simulink model "Trot"  (R2025b)
settings: Solver=VariableStepAuto  StartTime=0.0  StopTime=60  RelTol=0.01  AbsTol=0.01  EnableMultiTasking=on
undefined symbols (not defined in the file): a, b, c, X, Y, Z
libraries: sm_lib x58, nesl_utility x37, hdlsllib x12
(part 3 of 4)

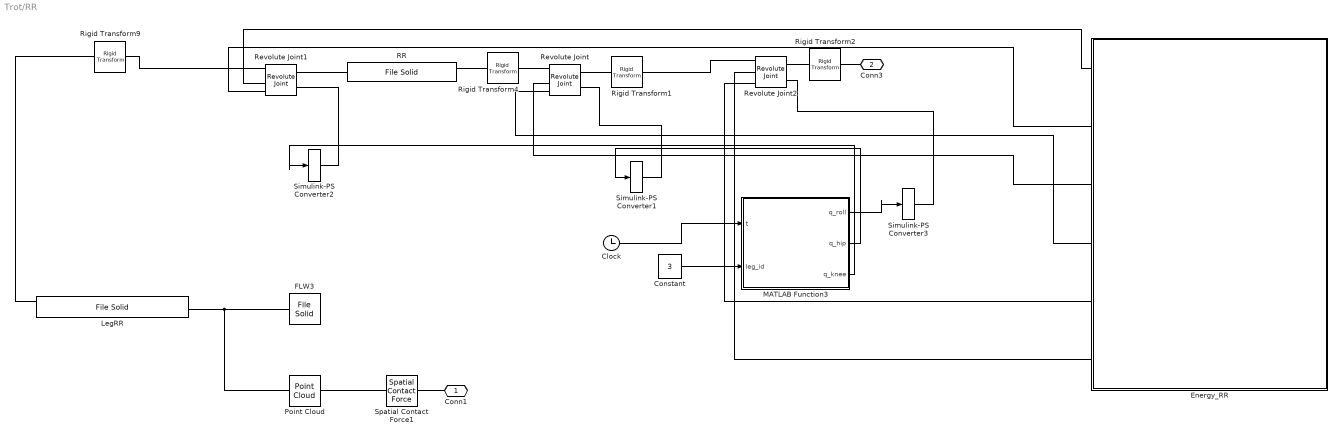
== system Trot/RR ==
  Clock : Clock
  Constant : Constant  Value=3
  Energy_RR : Subsystem
  FLW3 : sm_lib/Body Elements/File Solid  ExtGeomFileName=Cheng Shin C-166-1.stp  UnitType=FromFile  ExtGeomFileUnits=m  StepReaderType=HEX  ExportConvexHullGeometry=on  InertiaType=CalculateFromGeometry  BasedOnType=Density  Density=400  DensityUnits=kg/m^3  Mass=1  MassUnits=kg  CenterOfMass=[0 0 0]  CenterOfMassUnits=m  MomentsOfInertia=[1 1 1]  MomentsOfInertiaUnits=kg*m^2  ProductsOfInertia=[0 0 0]  ProductsOfInertiaUnits=kg*m^2  GraphicType=FromGeometry  MarkerShape=Sphere  MarkerSize=10  GraphicVisPropType=AdvancedVisualProperties  GraphicDiffuseColor=[0.1 0.1 0.1]  GraphicOpacity=1  GraphicSpecularColor=[0.2 0.2 0.2 1.0]  GraphicAmbientColor=[0.05 0.05 0.05 1.0]  GraphicEmissiveColor=[0.0 0.0 0.0 1.0]  GraphicShininess=10  DoExposeReferenceFrame=off  SerializedFrames=<Frames><Frame><Id>Frame1</Id><Value><Name>F1</Name><Origin><Source>CenterOfMassFrame</Source><FeatureName>toroidal surface 99</FeatureName></Origin><PrimaryAxis><DefinedDirection>+Z</DefinedDirection><Source>ReferenceFrame</Source><SourceDirection>+Z</SourceDirection><FeatureName></FeatureName></PrimaryAxis><SecondaryAxis><DefinedDirection>+X</DefinedDirection><Source>ReferenceFrame</Source><SourceDirection>+X</SourceDirection><FeatureName></FeatureName></SecondaryAxis></Value></Frame></Frames>
  LegRR : sm_lib/Body Elements/File Solid  ExtGeomFileName=leg.STEP  UnitType=FromFile  ExtGeomFileUnits=m  StepReaderType=HEX  ExportConvexHullGeometry=on  InertiaType=CalculateFromGeometry  BasedOnType=Density  Density=800  DensityUnits=kg/m^3  Mass=1  MassUnits=kg  CenterOfMass=[0 0 0]  CenterOfMassUnits=m  MomentsOfInertia=[1 1 1]  MomentsOfInertiaUnits=kg*m^2  ProductsOfInertia=[0 0 0]  ProductsOfInertiaUnits=kg*m^2  GraphicType=FromGeometry  MarkerShape=Sphere  MarkerSize=10  GraphicVisPropType=AdvancedVisualProperties  GraphicDiffuseColor=[0 0 0]  GraphicOpacity=1  GraphicSpecularColor=[0.9 0.9 0.9 1.0]  GraphicAmbientColor=[0.1 0.1 0.1 1.0]  GraphicEmissiveColor=[0.0 0.0 0.0 1.0]  GraphicShininess=100  DoExposeReferenceFrame=off  SerializedFrames=|
      | <Frames>
      | 
      |   <Frame>
      |     <Id>Frame1</Id>
      |     <Value>
      |       <Name>L-K link</Name>
      |       <Origin>
      |         <Source>GeometricFeature</Source>
      |         <FeatureName>cylindrical surface 6</FeatureName>
      |       </Origin>
      |       <PrimaryAxis>
      |         <DefinedDirection>+Z</DefinedDirection>
      |         <Source>ReferenceFrame</Source>
      |         <SourceDirection>+Z</SourceDirection>
      |         <FeatureName></FeatureName>
      |       </PrimaryAxis>
      |       <SecondaryAxis>
      |         <DefinedDirection>+X</DefinedDirection>
      |         <Source>ReferenceFrame</Source>
      |         <SourceDirection>-X</SourceDirection>
      |         <FeatureName></FeatureName>
      |       </SecondaryAxis>
      |     </Value>
      |   </Frame>
      | 
      |   <Frame>
      |     <Id>Frame2</Id>
      |     <Value>
      |       <Name>L-W link</Name>
      |       <Origin>
      |         <Source>GeometricFeature</Source>
      |         <FeatureName>cylindrical surface 4</FeatureName>
      |       </Origin>
      |       <PrimaryAxis>
      |         <DefinedDirection>+Z</DefinedDirection>
      |         <Source>ReferenceFrame</Source>
      |         <SourceDirection>+Z</SourceDirection>
      |         <FeatureName></FeatureName>
      |       </PrimaryAxis>
      |       <SecondaryAxis>
      |         <DefinedDirection>+X</DefinedDirection>
      |         <Source>ReferenceFrame</Source>
      |         <SourceDirection>-X</SourceDirection>
      |         <FeatureName></FeatureName>
      |       </SecondaryAxis>
      |     </Value>
      |   </Frame>
      | 
      | </Frames>
  MATLAB Function3 : MATLAB Function  TreatAsAtomicUnit=on
  Point Cloud : sm_lib/Curves and Surfaces/Point Cloud  CoordinatesMatrix=wheel_pts  CoordinatesMatrixUnits=m  GraphicType=MarkerCloud  GraphicSphereRadius=1e-2  GraphicSphereRadiusUnits=m  GraphicVisPropType=SimpleVisualProperties  GraphicDiffuseColor=[0.5 0.5 0.5]  GraphicOpacity=1  GraphicSpecularColor=[0.5 0.5 0.5 1.0]  GraphicAmbientColor=[0.15 0.15 0.15 1.0]  GraphicEmissiveColor=[0.0 0.0 0.0 1.0]  GraphicShininess=75
  RR : sm_lib/Body Elements/File Solid  ExtGeomFileName=haut patte D.STEP  UnitType=FromFile  ExtGeomFileUnits=m  StepReaderType=HEX  ExportConvexHullGeometry=on  InertiaType=CalculateFromGeometry  BasedOnType=Density  Density=800  DensityUnits=kg/m^3  Mass=1  MassUnits=kg  CenterOfMass=[0 0 0]  CenterOfMassUnits=m  MomentsOfInertia=[1 1 1]  MomentsOfInertiaUnits=kg*m^2  ProductsOfInertia=[0 0 0]  ProductsOfInertiaUnits=kg*m^2  GraphicType=FromGeometry  MarkerShape=Sphere  MarkerSize=10  GraphicVisPropType=AdvancedVisualProperties  GraphicDiffuseColor=[0.9 0.9 0.9]  GraphicOpacity=1  GraphicSpecularColor=[0.9 0.9 0.9 1.0]  GraphicAmbientColor=[0.1 0.1 0.1 1.0]  GraphicEmissiveColor=[0.0 0.0 0.0 1.0]  GraphicShininess=100  DoExposeReferenceFrame=off  SerializedFrames=<Frames><Frame><Id>Frame1</Id><Value><Name>H-L link</Name><Origin><Source>GeometricFeature</Source><FeatureName>spherical surface 2</FeatureName></Origin><PrimaryAxis><DefinedDirection>+Z</DefinedDirection><Source>ReferenceFrame</Source><SourceDirection>+Z</SourceDirection><FeatureName></FeatureName></PrimaryAxis><SecondaryAxis><DefinedDirection>+X</DefinedDirection><Source>ReferenceFrame</Source><SourceDirection>-Y</SourceDirection><FeatureName></FeatureName></SecondaryAxis></Value></Frame><Frame><Id>Frame2</Id><Value><Name>L-K link</Name><Origin><Source>GeometricFeature</Source><FeatureName>cylindrical surface 2</FeatureName></Origin><PrimaryAxis><DefinedDirection>+Z</DefinedDirection><Source>ReferenceFrame</Source><SourceDirection>+Z</SourceDirection><FeatureName></FeatureName></PrimaryAxis><SecondaryAxis><DefinedDirection>+X</DefinedDirection><Source>ReferenceFrame</Source><SourceDirection>-Y</SourceDirection><FeatureName></FeatureName></SecondaryAxis></Value></Frame></Frames>
  Revolute Joint : sm_lib/Joints/Revolute Joint  JointMode=Normal  CompositeWrenchDir=FollowerOnBase  CompositeWrenchFrame=BaseFrame  SenseConstraintForce=off  SenseConstraintTorque=off  SenseTotalForce=off  SenseTotalTorque=off  PositionTargetSpecify=off  PositionTargetPriority=High  PositionTargetValue=0  PositionTargetValueUnits=deg  VelocityTargetSpecify=off  VelocityTargetPriority=High  VelocityTargetValue=0  VelocityTargetValueUnits=deg/s  EquilibriumPosition=0  EquilibriumPositionUnits=deg  SpringStiffness=0  SpringStiffnessUnits=N*m/deg  DampingCoefficient=0  DampingCoefficientUnits=N*m/(deg/s)  LowerLimitSpecify=off  LowerLimitBound=-90  LowerLimitBoundUnits=deg  LowerLimitStiffness=1e4  LowerLimitStiffnessUnits=N*m/deg  LowerLimitDamping=10  LowerLimitDampingUnits=N*m/(deg/s)  LowerLimitTransitionRegionWidth=0.1  LowerLimitTransitionRegionWidthUnits=deg  UpperLimitSpecify=off  UpperLimitBound=90  UpperLimitBoundUnits=deg  UpperLimitStiffness=1e4  UpperLimitStiffnessUnits=N*m/deg  UpperLimitDamping=10  UpperLimitDampingUnits=N*m/(deg/s)  UpperLimitTransitionRegionWidth=0.1  UpperLimitTransitionRegionWidthUnits=deg  TorqueActuationMode=ComputedTorque  MotionActuationMode=InputMotion  SensePosition=on  SenseVelocity=on  SenseAcceleration=off  SenseTorqueForce=on  SenseLowerLimitTorqueForce=off  SenseUpperLimitTorqueForce=off
  Revolute Joint1 : sm_lib/Joints/Revolute Joint  JointMode=Normal  CompositeWrenchDir=FollowerOnBase  CompositeWrenchFrame=BaseFrame  SenseConstraintForce=off  SenseConstraintTorque=off  SenseTotalForce=off  SenseTotalTorque=off  PositionTargetSpecify=off  PositionTargetPriority=High  PositionTargetValue=0  PositionTargetValueUnits=deg  VelocityTargetSpecify=off  VelocityTargetPriority=High  VelocityTargetValue=0  VelocityTargetValueUnits=deg/s  EquilibriumPosition=0  EquilibriumPositionUnits=deg  SpringStiffness=0  SpringStiffnessUnits=N*m/deg  DampingCoefficient=0  DampingCoefficientUnits=N*m/(deg/s)  LowerLimitSpecify=off  LowerLimitBound=-90  LowerLimitBoundUnits=deg  LowerLimitStiffness=1e4  LowerLimitStiffnessUnits=N*m/deg  LowerLimitDamping=10  LowerLimitDampingUnits=N*m/(deg/s)  LowerLimitTransitionRegionWidth=0.1  LowerLimitTransitionRegionWidthUnits=deg  UpperLimitSpecify=off  UpperLimitBound=90  UpperLimitBoundUnits=deg  UpperLimitStiffness=1e4  UpperLimitStiffnessUnits=N*m/deg  UpperLimitDamping=10  UpperLimitDampingUnits=N*m/(deg/s)  UpperLimitTransitionRegionWidth=0.1  UpperLimitTransitionRegionWidthUnits=deg  TorqueActuationMode=ComputedTorque  MotionActuationMode=InputMotion  SensePosition=on  SenseVelocity=on  SenseAcceleration=off  SenseTorqueForce=on  SenseLowerLimitTorqueForce=off  SenseUpperLimitTorqueForce=off
  Revolute Joint2 : sm_lib/Joints/Revolute Joint  JointMode=Normal  CompositeWrenchDir=FollowerOnBase  CompositeWrenchFrame=BaseFrame  SenseConstraintForce=off  SenseConstraintTorque=off  SenseTotalForce=off  SenseTotalTorque=off  PositionTargetSpecify=off  PositionTargetPriority=High  PositionTargetValue=0  PositionTargetValueUnits=deg  VelocityTargetSpecify=off  VelocityTargetPriority=High  VelocityTargetValue=0  VelocityTargetValueUnits=deg/s  EquilibriumPosition=0  EquilibriumPositionUnits=deg  SpringStiffness=0  SpringStiffnessUnits=N*m/deg  DampingCoefficient=0  DampingCoefficientUnits=N*m/(deg/s)  LowerLimitSpecify=off  LowerLimitBound=-90  LowerLimitBoundUnits=deg  LowerLimitStiffness=1e4  LowerLimitStiffnessUnits=N*m/deg  LowerLimitDamping=10  LowerLimitDampingUnits=N*m/(deg/s)  LowerLimitTransitionRegionWidth=0.1  LowerLimitTransitionRegionWidthUnits=deg  UpperLimitSpecify=off  UpperLimitBound=90  UpperLimitBoundUnits=deg  UpperLimitStiffness=1e4  UpperLimitStiffnessUnits=N*m/deg  UpperLimitDamping=10  UpperLimitDampingUnits=N*m/(deg/s)  UpperLimitTransitionRegionWidth=0.1  UpperLimitTransitionRegionWidthUnits=deg  TorqueActuationMode=ComputedTorque  MotionActuationMode=InputMotion  SensePosition=on  SenseVelocity=on  SenseAcceleration=off  SenseTorqueForce=off  SenseLowerLimitTorqueForce=off  SenseUpperLimitTorqueForce=off
  Rigid Transform1 : sm_lib/Frames and Transforms/Rigid Transform  RotationMethod=AlignedAxes  FollAlignAxisA=+Z  BaseAlignAxisA=+Y  FollAlignAxisB=+X  BaseAlignAxisB=+X  RotationStandardAxis=+Z  RotationAngle=0  RotationAngleUnits=deg  RotationArbitraryAxis=[0 0 1]  RotationSequenceAxes=FollowerAxes  RotationSequence=XYX  RotationSequenceAngles=[0 0 0]  RotationSequenceAnglesUnits=deg  RotationMatrix=[1 0 0;0 1 0;0 0 1]  Quaternion=[1 0 0 0]  TranslationMethod=None  TranslationCartesianOffset=[0 0 0]  TranslationCartesianOffsetUnits=m  TranslationStandardAxis=+Z  TranslationStandardOffset=0  TranslationStandardOffsetUnits=m  TranslationROffset=0  TranslationROffsetUnits=m  TranslationThetaOffset=0  TranslationThetaOffsetUnits=deg  TranslationZOffset=0  TranslationZOffsetUnits=m
  Rigid Transform2 : sm_lib/Frames and Transforms/Rigid Transform  RotationMethod=AlignedAxes  FollAlignAxisA=+Y  BaseAlignAxisA=+Y  FollAlignAxisB=+Z  BaseAlignAxisB=+X  RotationStandardAxis=+Z  RotationAngle=0  RotationAngleUnits=deg  RotationArbitraryAxis=[0 0 1]  RotationSequenceAxes=FollowerAxes  RotationSequence=XYX  RotationSequenceAngles=[0 0 0]  RotationSequenceAnglesUnits=deg  RotationMatrix=[1 0 0;0 1 0;0 0 1]  Quaternion=[1 0 0 0]  TranslationMethod=None  TranslationCartesianOffset=[0 0 0]  TranslationCartesianOffsetUnits=m  TranslationStandardAxis=+Z  TranslationStandardOffset=0  TranslationStandardOffsetUnits=m  TranslationROffset=0  TranslationROffsetUnits=m  TranslationThetaOffset=0  TranslationThetaOffsetUnits=deg  TranslationZOffset=0  TranslationZOffsetUnits=m
  Rigid Transform4 : sm_lib/Frames and Transforms/Rigid Transform  RotationMethod=RotationSequence  FollAlignAxisA=+X  BaseAlignAxisA=+Y  FollAlignAxisB=+Y  BaseAlignAxisB=+Z  RotationStandardAxis=+Z  RotationAngle=0  RotationAngleUnits=deg  RotationArbitraryAxis=[0 0 1]  RotationSequenceAxes=FollowerAxes  RotationSequence=XYZ  RotationSequenceAngles=[0 0 -60]  RotationSequenceAnglesUnits=deg  RotationMatrix=[1 0 0;0 1 0;0 0 1]  Quaternion=[1 0 0 0]  TranslationMethod=None  TranslationCartesianOffset=[0 0 0]  TranslationCartesianOffsetUnits=m  TranslationStandardAxis=+Z  TranslationStandardOffset=0  TranslationStandardOffsetUnits=m  TranslationROffset=0  TranslationROffsetUnits=m  TranslationThetaOffset=0  TranslationThetaOffsetUnits=deg  TranslationZOffset=0  TranslationZOffsetUnits=m
  Rigid Transform9 : sm_lib/Frames and Transforms/Rigid Transform  RotationMethod=RotationSequence  FollAlignAxisA=+X  BaseAlignAxisA=+Y  FollAlignAxisB=+Y  BaseAlignAxisB=+Z  RotationStandardAxis=+Z  RotationAngle=0  RotationAngleUnits=deg  RotationArbitraryAxis=[0 0 1]  RotationSequenceAxes=FollowerAxes  RotationSequence=XYZ  RotationSequenceAngles=[0 0 -30]  RotationSequenceAnglesUnits=deg  RotationMatrix=[1 0 0;0 1 0;0 0 1]  Quaternion=[1 0 0 0]  TranslationMethod=None  TranslationCartesianOffset=[0 0 0]  TranslationCartesianOffsetUnits=m  TranslationStandardAxis=+Z  TranslationStandardOffset=0  TranslationStandardOffsetUnits=m  TranslationROffset=0  TranslationROffsetUnits=m  TranslationThetaOffset=0  TranslationThetaOffsetUnits=deg  TranslationZOffset=0  TranslationZOffsetUnits=m
  Simulink-PS Converter1 : nesl_utility/Simulink-PS Converter  PhysicalDomain=network_engine_domain  SubClassName=ps_input  LeftPortType=input  RightPortType=output  PseudoPeriodic=off  Frequencies=[]  NoiseDistribution=none  NoiseParameters=[]  Unit=1  AffineConversion=off  FilteringAndDerivatives=filter  SimscapeFilterOrder=2  InputFilterTimeConstant=0.001  UdotUserProvided=0
  Simulink-PS Converter2 : nesl_utility/Simulink-PS Converter  PhysicalDomain=network_engine_domain  SubClassName=ps_input  LeftPortType=input  RightPortType=output  PseudoPeriodic=off  Frequencies=[]  NoiseDistribution=none  NoiseParameters=[]  Unit=1  AffineConversion=off  FilteringAndDerivatives=filter  SimscapeFilterOrder=2  InputFilterTimeConstant=0.001  UdotUserProvided=0
  Simulink-PS Converter3 : nesl_utility/Simulink-PS Converter  PhysicalDomain=network_engine_domain  SubClassName=ps_input  LeftPortType=input  RightPortType=output  PseudoPeriodic=off  Frequencies=[]  NoiseDistribution=none  NoiseParameters=[]  Unit=1  AffineConversion=off  FilteringAndDerivatives=filter  SimscapeFilterOrder=2  InputFilterTimeConstant=0.001  UdotUserProvided=0
  Spatial Contact Force1 : sm_lib/Forces and Torques/Spatial Contact Force  SenseSeparationDistance=off  NormalForceType=SmoothSpringDamper  NormalStiffness=10e5  NormalStiffnessUnits=N/m  NormalDamping=10e3  NormalDampingUnits=N/(m/s)  NormalTransitionRegionWidth=0.6  NormalTransitionRegionWidthUnits=m  FrictionType=SmoothStickSlip  CoefficientOfStaticFriction=0.9  CoefficientOfDynamicFriction=0.7  FrictionalCriticalVelocity=1e-3  FrictionalCriticalVelocityUnits=m/s  SenseContactSignal=off  SensePenetrationDepth=off  SenseNormalVelocity=off  SenseTangentialVelocity=off  SensingForceTorqueDirection=BaseOnFollower  SensingForceTorqueResolutionFrame=ContactFrame  SenseNormalForce=off  SenseNormalForceMagnitude=off  SenseNormalTorque=off  SenseFrictionalForce=off  SenseFrictionalForceMagnitude=off  SenseFrictionalTorque=off  SenseTotalForce=off  SenseTotalTorque=off  SenseContactBaseRotation=off  SenseContactBaseTranslation=off  SenseContactFollowerRotation=off  SenseContactFollowerTranslation=off  ZeroCrossDetectContactStartAndEnd=off
  Conn1 : PMIOPort  Side=Left
  Conn3 : PMIOPort  Port=2  Side=Right
  wires:
  MATLAB Function3/1(q_roll) -> Simulink-PS Converter3/1
  Constant/1 -> MATLAB Function3/2(leg_id)
  Clock/1 -> MATLAB Function3/1(t)
  MATLAB Function3/2(q_hip) -> Simulink-PS Converter1/1
  MATLAB Function3/3(q_knee) -> Simulink-PS Converter2/1
  connections:
  Rigid Transform1/RConn1 -- Revolute Joint/LConn1
  Rigid Transform4/LConn1 -- Revolute Joint/RConn1
  Rigid Transform1/LConn1 -- Revolute Joint2/RConn1
  Spatial Contact Force1/LConn1 -- Conn1/RConn1
  LegRR/RConn1 -- Point Cloud/LConn1 -- FLW3/LConn1
  Rigid Transform4/RConn1 -- RR/LConn1
  Revolute Joint1/LConn1 -- RR/RConn1
  Rigid Transform9/LConn1 -- Revolute Joint1/RConn1
  LegRR/LConn1 -- Rigid Transform9/RConn1
  Rigid Transform2/LConn1 -- Conn3/RConn1
  Simulink-PS Converter3/RConn1 -- Revolute Joint2/LConn2
  Simulink-PS Converter1/RConn1 -- Revolute Joint/LConn2
  Revolute Joint1/LConn2 -- Simulink-PS Converter2/RConn1
  Revolute Joint2/LConn1 -- Rigid Transform2/RConn1
  Point Cloud/RConn1 -- Spatial Contact Force1/RConn1
  Revolute Joint1/RConn3 -- Energy_RR/LConn1
  Revolute Joint1/RConn4 -- Energy_RR/LConn2
  Revolute Joint/RConn3 -- Energy_RR/LConn3
  Revolute Joint/RConn4 -- Energy_RR/LConn4
  Revolute Joint2/RConn3 -- Energy_RR/LConn5
  Revolute Joint2/RConn2 -- Energy_RR/LConn6

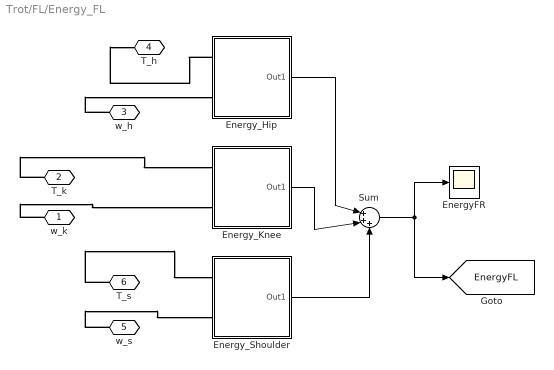
== system Trot/FL/Energy_FL ==
  EnergyFR : Scope
  Energy_Hip : Subsystem
  Energy_Knee : Subsystem
  Energy_Shoulder : Subsystem
  Sum : Sum  Inputs=|+++
  w_k : PMIOPort  Side=Left
  T_k : PMIOPort  Port=2  Side=Left
  w_h : PMIOPort  Port=3  Side=Left
  T_h : PMIOPort  Port=4  Side=Left
  w_s : PMIOPort  Port=5  Side=Left
  T_s : PMIOPort  Port=6  Side=Left
  tag scope: EnergyFL=global
  wires:
  Sum/1 -> [EnergyFL], EnergyFR/1
  Energy_Hip/1(Out1) -> Sum/1
  Energy_Shoulder/1(Out1) -> Sum/3
  Energy_Knee/1(Out1) -> Sum/2
  connections:
  T_k/RConn1 -- Energy_Knee/LConn1
  w_s/RConn1 -- Energy_Shoulder/LConn2
  w_h/RConn1 -- Energy_Hip/LConn2
  w_k/RConn1 -- Energy_Knee/LConn2
  Energy_Hip/LConn1 -- T_h/RConn1
  T_s/RConn1 -- Energy_Shoulder/LConn1

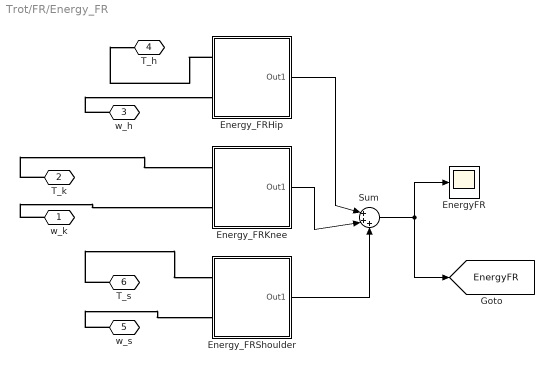
== system Trot/FR/Energy_FR ==
  EnergyFR : Scope
  Energy_FRHip : Subsystem
  Energy_FRKnee : Subsystem
  Energy_FRShoulder : Subsystem
  Sum : Sum  Inputs=|+++
  w_k : PMIOPort  Side=Left
  T_k : PMIOPort  Port=2  Side=Left
  w_h : PMIOPort  Port=3  Side=Left
  T_h : PMIOPort  Port=4  Side=Left
  w_s : PMIOPort  Port=5  Side=Left
  T_s : PMIOPort  Port=6  Side=Left
  tag scope: EnergyFR=global
  wires:
  Sum/1 -> [EnergyFR], EnergyFR/1
  Energy_FRHip/1(Out1) -> Sum/1
  Energy_FRShoulder/1(Out1) -> Sum/3
  Energy_FRKnee/1(Out1) -> Sum/2
  connections:
  T_k/RConn1 -- Energy_FRKnee/LConn1
  w_s/RConn1 -- Energy_FRShoulder/LConn2
  w_h/RConn1 -- Energy_FRHip/LConn2
  w_k/RConn1 -- Energy_FRKnee/LConn2
  Energy_FRHip/LConn1 -- T_h/RConn1
  T_s/RConn1 -- Energy_FRShoulder/LConn1

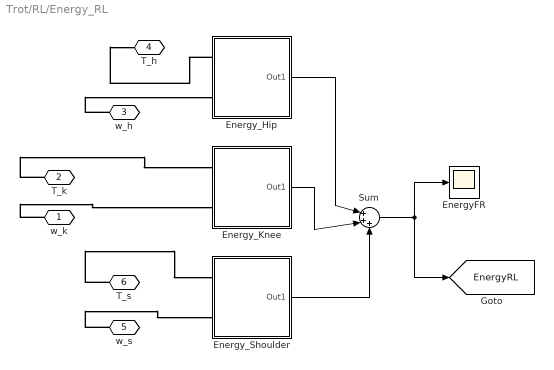
== system Trot/RL/Energy_RL ==
  EnergyFR : Scope
  Energy_Hip : Subsystem
  Energy_Knee : Subsystem
  Energy_Shoulder : Subsystem
  Sum : Sum  Inputs=|+++
  w_k : PMIOPort  Side=Left
  T_k : PMIOPort  Port=2  Side=Left
  w_h : PMIOPort  Port=3  Side=Left
  T_h : PMIOPort  Port=4  Side=Left
  w_s : PMIOPort  Port=5  Side=Left
  T_s : PMIOPort  Port=6  Side=Left
  tag scope: EnergyRL=global
  wires:
  Sum/1 -> [EnergyRL], EnergyFR/1
  Energy_Hip/1(Out1) -> Sum/1
  Energy_Shoulder/1(Out1) -> Sum/3
  Energy_Knee/1(Out1) -> Sum/2
  connections:
  T_k/RConn1 -- Energy_Knee/LConn1
  w_s/RConn1 -- Energy_Shoulder/LConn2
  w_h/RConn1 -- Energy_Hip/LConn2
  w_k/RConn1 -- Energy_Knee/LConn2
  Energy_Hip/LConn1 -- T_h/RConn1
  T_s/RConn1 -- Energy_Shoulder/LConn1

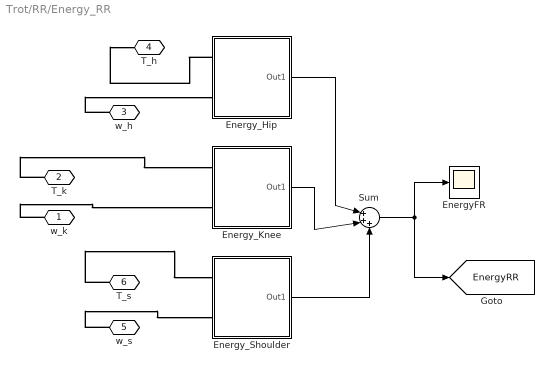
== system Trot/RR/Energy_RR ==
  EnergyFR : Scope
  Energy_Hip : Subsystem
  Energy_Knee : Subsystem
  Energy_Shoulder : Subsystem
  Sum : Sum  Inputs=|+++
  w_k : PMIOPort  Side=Left
  T_k : PMIOPort  Port=2  Side=Left
  w_h : PMIOPort  Port=3  Side=Left
  T_h : PMIOPort  Port=4  Side=Left
  w_s : PMIOPort  Port=5  Side=Left
  T_s : PMIOPort  Port=6  Side=Left
  tag scope: EnergyRR=global
  wires:
  Sum/1 -> [EnergyRR], EnergyFR/1
  Energy_Hip/1(Out1) -> Sum/1
  Energy_Shoulder/1(Out1) -> Sum/3
  Energy_Knee/1(Out1) -> Sum/2
  connections:
  T_k/RConn1 -- Energy_Knee/LConn1
  w_s/RConn1 -- Energy_Shoulder/LConn2
  w_h/RConn1 -- Energy_Hip/LConn2
  w_k/RConn1 -- Energy_Knee/LConn2
  Energy_Hip/LConn1 -- T_h/RConn1
  T_s/RConn1 -- Energy_Shoulder/LConn1

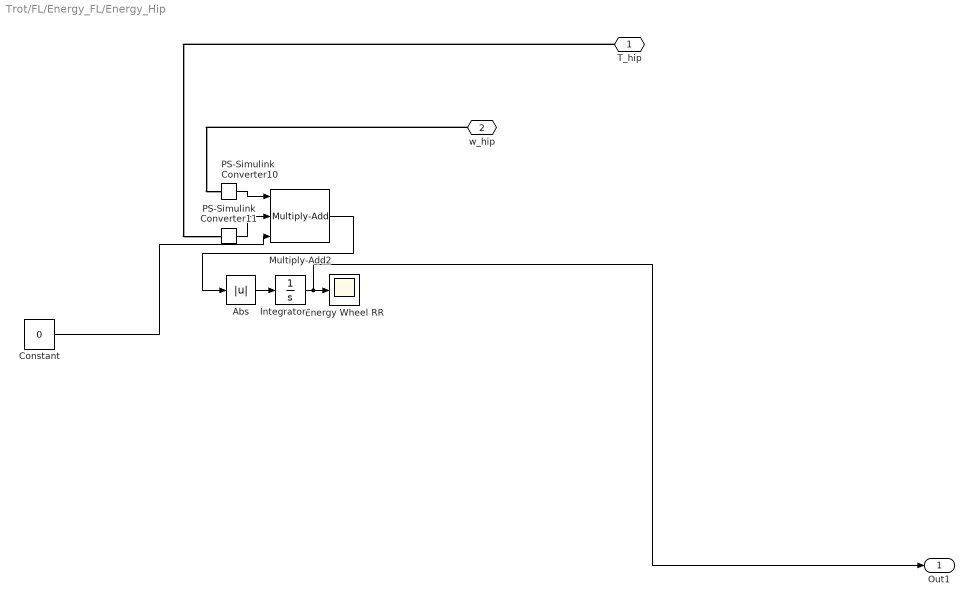
== system Trot/FL/Energy_FL/Energy_Hip ==
  Abs : Abs  SaturateOnIntegerOverflow=off
  Constant : Constant  Value=0
  Energy Wheel RR : Scope
      settings: ActiveDisplayYMinimum=-137.61876169666837  ActiveDisplayYMaximum=1238.5688552700155  DataLoggingVariableName=ScopeData3
  Integrator : Integrator
  Multiply-Add2 : hdlsllib/HDL Operations/Multiply-Add  Function=c+(a.*b)  datatype=Inherit: Inherit via internal rule  DoSatur=off  FMA=off
  PS-Simulink Converter10 : nesl_utility/PS-Simulink Converter  PhysicalDomain=network_engine_domain  SubClassName=ps_output  LeftPortType=input  RightPortType=output  PseudoPeriodic=off  Frequencies=[]  VectorFormat=inherit  Unit=inherit  AffineConversion=off
  PS-Simulink Converter11 : nesl_utility/PS-Simulink Converter  PhysicalDomain=network_engine_domain  SubClassName=ps_output  LeftPortType=input  RightPortType=output  PseudoPeriodic=off  Frequencies=[]  VectorFormat=inherit  Unit=inherit  AffineConversion=off
  T_hip : PMIOPort  Side=Left
  w_hip : PMIOPort  Port=2  Side=Left
  Out1 : Outport
  wires:
  PS-Simulink Converter10/1 -> Multiply-Add2/1
  Integrator/1 -> Out1/1, Energy Wheel RR/1
  PS-Simulink Converter11/1 -> Multiply-Add2/2
  Constant/1 -> Multiply-Add2/3
  Abs/1 -> Integrator/1
  Multiply-Add2/1 -> Abs/1
  connections:
  T_hip/RConn1 -- PS-Simulink Converter11/LConn1
  w_hip/RConn1 -- PS-Simulink Converter10/LConn1

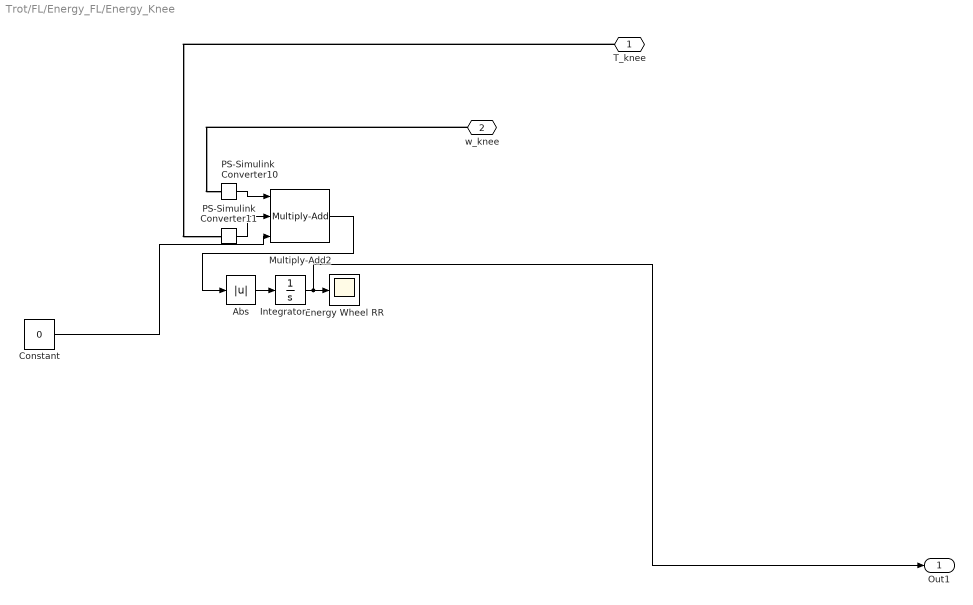
== system Trot/FL/Energy_FL/Energy_Knee ==
  Abs : Abs  SaturateOnIntegerOverflow=off
  Constant : Constant  Value=0
  Energy Wheel RR : Scope
      settings: ActiveDisplayYMinimum=-137.61876169666837  ActiveDisplayYMaximum=1238.5688552700155  DataLoggingVariableName=ScopeData3
  Integrator : Integrator
  Multiply-Add2 : hdlsllib/HDL Operations/Multiply-Add  Function=c+(a.*b)  datatype=Inherit: Inherit via internal rule  DoSatur=off  FMA=off
  PS-Simulink Converter10 : nesl_utility/PS-Simulink Converter  PhysicalDomain=network_engine_domain  SubClassName=ps_output  LeftPortType=input  RightPortType=output  PseudoPeriodic=off  Frequencies=[]  VectorFormat=inherit  Unit=inherit  AffineConversion=off
  PS-Simulink Converter11 : nesl_utility/PS-Simulink Converter  PhysicalDomain=network_engine_domain  SubClassName=ps_output  LeftPortType=input  RightPortType=output  PseudoPeriodic=off  Frequencies=[]  VectorFormat=inherit  Unit=inherit  AffineConversion=off
  T_knee : PMIOPort  Side=Left
  w_knee : PMIOPort  Port=2  Side=Left
  Out1 : Outport
  wires:
  Multiply-Add2/1 -> Abs/1
  Abs/1 -> Integrator/1
  Constant/1 -> Multiply-Add2/3
  PS-Simulink Converter11/1 -> Multiply-Add2/2
  Integrator/1 -> Energy Wheel RR/1, Out1/1
  PS-Simulink Converter10/1 -> Multiply-Add2/1
  connections:
  w_knee/RConn1 -- PS-Simulink Converter10/LConn1
  T_knee/RConn1 -- PS-Simulink Converter11/LConn1

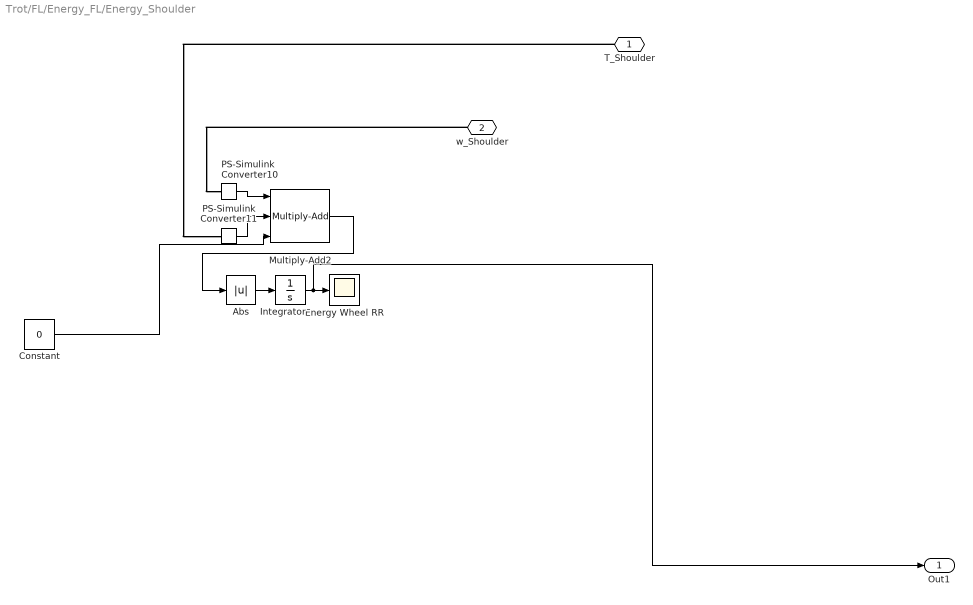
== system Trot/FL/Energy_FL/Energy_Shoulder ==
  Abs : Abs  SaturateOnIntegerOverflow=off
  Constant : Constant  Value=0
  Energy Wheel RR : Scope
      settings: ActiveDisplayYMinimum=-137.61876169666837  ActiveDisplayYMaximum=1238.5688552700155  DataLoggingVariableName=ScopeData3
  Integrator : Integrator
  Multiply-Add2 : hdlsllib/HDL Operations/Multiply-Add  Function=c+(a.*b)  datatype=Inherit: Inherit via internal rule  DoSatur=off  FMA=off
  PS-Simulink Converter10 : nesl_utility/PS-Simulink Converter  PhysicalDomain=network_engine_domain  SubClassName=ps_output  LeftPortType=input  RightPortType=output  PseudoPeriodic=off  Frequencies=[]  VectorFormat=inherit  Unit=inherit  AffineConversion=off
  PS-Simulink Converter11 : nesl_utility/PS-Simulink Converter  PhysicalDomain=network_engine_domain  SubClassName=ps_output  LeftPortType=input  RightPortType=output  PseudoPeriodic=off  Frequencies=[]  VectorFormat=inherit  Unit=inherit  AffineConversion=off
  T_Shoulder : PMIOPort  Side=Left
  w_Shoulder : PMIOPort  Port=2  Side=Left
  Out1 : Outport
  wires:
  PS-Simulink Converter10/1 -> Multiply-Add2/1
  Integrator/1 -> Out1/1, Energy Wheel RR/1
  PS-Simulink Converter11/1 -> Multiply-Add2/2
  Constant/1 -> Multiply-Add2/3
  Abs/1 -> Integrator/1
  Multiply-Add2/1 -> Abs/1
  connections:
  T_Shoulder/RConn1 -- PS-Simulink Converter11/LConn1
  w_Shoulder/RConn1 -- PS-Simulink Converter10/LConn1

== system Trot/FR/Energy_FR/Energy_FRHip ==
  Abs : Abs  SaturateOnIntegerOverflow=off
  Constant : Constant  Value=0
  Energy Wheel RR : Scope
      settings: ActiveDisplayYMinimum=-137.61876169666837  ActiveDisplayYMaximum=1238.5688552700155  DataLoggingVariableName=ScopeData3
  Integrator : Integrator
  Multiply-Add2 : hdlsllib/HDL Operations/Multiply-Add  Function=c+(a.*b)  datatype=Inherit: Inherit via internal rule  DoSatur=off  FMA=off
  PS-Simulink Converter10 : nesl_utility/PS-Simulink Converter  PhysicalDomain=network_engine_domain  SubClassName=ps_output  LeftPortType=input  RightPortType=output  PseudoPeriodic=off  Frequencies=[]  VectorFormat=inherit  Unit=inherit  AffineConversion=off
  PS-Simulink Converter11 : nesl_utility/PS-Simulink Converter  PhysicalDomain=network_engine_domain  SubClassName=ps_output  LeftPortType=input  RightPortType=output  PseudoPeriodic=off  Frequencies=[]  VectorFormat=inherit  Unit=inherit  AffineConversion=off
  T_hip : PMIOPort  Side=Left
  w_hip : PMIOPort  Port=2  Side=Left
  Out1 : Outport
  wires:
  PS-Simulink Converter10/1 -> Multiply-Add2/1
  Integrator/1 -> Out1/1, Energy Wheel RR/1
  PS-Simulink Converter11/1 -> Multiply-Add2/2
  Constant/1 -> Multiply-Add2/3
  Abs/1 -> Integrator/1
  Multiply-Add2/1 -> Abs/1
  connections:
  T_hip/RConn1 -- PS-Simulink Converter11/LConn1
  w_hip/RConn1 -- PS-Simulink Converter10/LConn1

== system Trot/FR/Energy_FR/Energy_FRKnee ==
  Abs : Abs  SaturateOnIntegerOverflow=off
  Constant : Constant  Value=0
  Energy Wheel RR : Scope
      settings: ActiveDisplayYMinimum=-137.61876169666837  ActiveDisplayYMaximum=1238.5688552700155  DataLoggingVariableName=ScopeData3
  Integrator : Integrator
  Multiply-Add2 : hdlsllib/HDL Operations/Multiply-Add  Function=c+(a.*b)  datatype=Inherit: Inherit via internal rule  DoSatur=off  FMA=off
  PS-Simulink Converter10 : nesl_utility/PS-Simulink Converter  PhysicalDomain=network_engine_domain  SubClassName=ps_output  LeftPortType=input  RightPortType=output  PseudoPeriodic=off  Frequencies=[]  VectorFormat=inherit  Unit=inherit  AffineConversion=off
  PS-Simulink Converter11 : nesl_utility/PS-Simulink Converter  PhysicalDomain=network_engine_domain  SubClassName=ps_output  LeftPortType=input  RightPortType=output  PseudoPeriodic=off  Frequencies=[]  VectorFormat=inherit  Unit=inherit  AffineConversion=off
  T_knee : PMIOPort  Side=Left
  w_knee : PMIOPort  Port=2  Side=Left
  Out1 : Outport
  wires:
  Multiply-Add2/1 -> Abs/1
  Abs/1 -> Integrator/1
  Constant/1 -> Multiply-Add2/3
  PS-Simulink Converter11/1 -> Multiply-Add2/2
  Integrator/1 -> Energy Wheel RR/1, Out1/1
  PS-Simulink Converter10/1 -> Multiply-Add2/1
  connections:
  w_knee/RConn1 -- PS-Simulink Converter10/LConn1
  T_knee/RConn1 -- PS-Simulink Converter11/LConn1

== system Trot/FR/Energy_FR/Energy_FRShoulder ==
  Abs : Abs  SaturateOnIntegerOverflow=off
  Constant : Constant  Value=0
  Energy Wheel RR : Scope
      settings: ActiveDisplayYMinimum=-137.61876169666837  ActiveDisplayYMaximum=1238.5688552700155  DataLoggingVariableName=ScopeData3
  Integrator : Integrator
  Multiply-Add2 : hdlsllib/HDL Operations/Multiply-Add  Function=c+(a.*b)  datatype=Inherit: Inherit via internal rule  DoSatur=off  FMA=off
  PS-Simulink Converter10 : nesl_utility/PS-Simulink Converter  PhysicalDomain=network_engine_domain  SubClassName=ps_output  LeftPortType=input  RightPortType=output  PseudoPeriodic=off  Frequencies=[]  VectorFormat=inherit  Unit=inherit  AffineConversion=off
  PS-Simulink Converter11 : nesl_utility/PS-Simulink Converter  PhysicalDomain=network_engine_domain  SubClassName=ps_output  LeftPortType=input  RightPortType=output  PseudoPeriodic=off  Frequencies=[]  VectorFormat=inherit  Unit=inherit  AffineConversion=off
  T_Shoulder : PMIOPort  Side=Left
  w_Shoulder : PMIOPort  Port=2  Side=Left
  Out1 : Outport
  wires:
  PS-Simulink Converter10/1 -> Multiply-Add2/1
  Integrator/1 -> Out1/1, Energy Wheel RR/1
  PS-Simulink Converter11/1 -> Multiply-Add2/2
  Constant/1 -> Multiply-Add2/3
  Abs/1 -> Integrator/1
  Multiply-Add2/1 -> Abs/1
  connections:
  T_Shoulder/RConn1 -- PS-Simulink Converter11/LConn1
  w_Shoulder/RConn1 -- PS-Simulink Converter10/LConn1

== system Trot/RL/Energy_RL/Energy_Hip ==
  Abs : Abs  SaturateOnIntegerOverflow=off
  Constant : Constant  Value=0
  Energy Wheel RR : Scope
      settings: ActiveDisplayYMinimum=-137.61876169666837  ActiveDisplayYMaximum=1238.5688552700155  DataLoggingVariableName=ScopeData3
  Integrator : Integrator
  Multiply-Add2 : hdlsllib/HDL Operations/Multiply-Add  Function=c+(a.*b)  datatype=Inherit: Inherit via internal rule  DoSatur=off  FMA=off
  PS-Simulink Converter10 : nesl_utility/PS-Simulink Converter  PhysicalDomain=network_engine_domain  SubClassName=ps_output  LeftPortType=input  RightPortType=output  PseudoPeriodic=off  Frequencies=[]  VectorFormat=inherit  Unit=inherit  AffineConversion=off
  PS-Simulink Converter11 : nesl_utility/PS-Simulink Converter  PhysicalDomain=network_engine_domain  SubClassName=ps_output  LeftPortType=input  RightPortType=output  PseudoPeriodic=off  Frequencies=[]  VectorFormat=inherit  Unit=inherit  AffineConversion=off
  T_hip : PMIOPort  Side=Left
  w_hip : PMIOPort  Port=2  Side=Left
  Out1 : Outport
  wires:
  PS-Simulink Converter10/1 -> Multiply-Add2/1
  Integrator/1 -> Out1/1, Energy Wheel RR/1
  PS-Simulink Converter11/1 -> Multiply-Add2/2
  Constant/1 -> Multiply-Add2/3
  Abs/1 -> Integrator/1
  Multiply-Add2/1 -> Abs/1
  connections:
  T_hip/RConn1 -- PS-Simulink Converter11/LConn1
  w_hip/RConn1 -- PS-Simulink Converter10/LConn1

== system Trot/RL/Energy_RL/Energy_Knee ==
  Abs : Abs  SaturateOnIntegerOverflow=off
  Constant : Constant  Value=0
  Energy Wheel RR : Scope
      settings: ActiveDisplayYMinimum=-137.61876169666837  ActiveDisplayYMaximum=1238.5688552700155  DataLoggingVariableName=ScopeData3
  Integrator : Integrator
  Multiply-Add2 : hdlsllib/HDL Operations/Multiply-Add  Function=c+(a.*b)  datatype=Inherit: Inherit via internal rule  DoSatur=off  FMA=off
  PS-Simulink Converter10 : nesl_utility/PS-Simulink Converter  PhysicalDomain=network_engine_domain  SubClassName=ps_output  LeftPortType=input  RightPortType=output  PseudoPeriodic=off  Frequencies=[]  VectorFormat=inherit  Unit=inherit  AffineConversion=off
  PS-Simulink Converter11 : nesl_utility/PS-Simulink Converter  PhysicalDomain=network_engine_domain  SubClassName=ps_output  LeftPortType=input  RightPortType=output  PseudoPeriodic=off  Frequencies=[]  VectorFormat=inherit  Unit=inherit  AffineConversion=off
  T_knee : PMIOPort  Side=Left
  w_knee : PMIOPort  Port=2  Side=Left
  Out1 : Outport
  wires:
  Multiply-Add2/1 -> Abs/1
  Abs/1 -> Integrator/1
  Constant/1 -> Multiply-Add2/3
  PS-Simulink Converter11/1 -> Multiply-Add2/2
  Integrator/1 -> Energy Wheel RR/1, Out1/1
  PS-Simulink Converter10/1 -> Multiply-Add2/1
  connections:
  w_knee/RConn1 -- PS-Simulink Converter10/LConn1
  T_knee/RConn1 -- PS-Simulink Converter11/LConn1

== system Trot/RL/Energy_RL/Energy_Shoulder ==
  Abs : Abs  SaturateOnIntegerOverflow=off
  Constant : Constant  Value=0
  Energy Wheel RR : Scope
      settings: ActiveDisplayYMinimum=-137.61876169666837  ActiveDisplayYMaximum=1238.5688552700155  DataLoggingVariableName=ScopeData3
  Integrator : Integrator
  Multiply-Add2 : hdlsllib/HDL Operations/Multiply-Add  Function=c+(a.*b)  datatype=Inherit: Inherit via internal rule  DoSatur=off  FMA=off
  PS-Simulink Converter10 : nesl_utility/PS-Simulink Converter  PhysicalDomain=network_engine_domain  SubClassName=ps_output  LeftPortType=input  RightPortType=output  PseudoPeriodic=off  Frequencies=[]  VectorFormat=inherit  Unit=inherit  AffineConversion=off
  PS-Simulink Converter11 : nesl_utility/PS-Simulink Converter  PhysicalDomain=network_engine_domain  SubClassName=ps_output  LeftPortType=input  RightPortType=output  PseudoPeriodic=off  Frequencies=[]  VectorFormat=inherit  Unit=inherit  AffineConversion=off
  T_Shoulder : PMIOPort  Side=Left
  w_Shoulder : PMIOPort  Port=2  Side=Left
  Out1 : Outport
  wires:
  PS-Simulink Converter10/1 -> Multiply-Add2/1
  Integrator/1 -> Out1/1, Energy Wheel RR/1
  PS-Simulink Converter11/1 -> Multiply-Add2/2
  Constant/1 -> Multiply-Add2/3
  Abs/1 -> Integrator/1
  Multiply-Add2/1 -> Abs/1
  connections:
  T_Shoulder/RConn1 -- PS-Simulink Converter11/LConn1
  w_Shoulder/RConn1 -- PS-Simulink Converter10/LConn1

== system Trot/RR/Energy_RR/Energy_Hip ==
  Abs : Abs  SaturateOnIntegerOverflow=off
  Constant : Constant  Value=0
  Energy Wheel RR : Scope
      settings: ActiveDisplayYMinimum=-137.61876169666837  ActiveDisplayYMaximum=1238.5688552700155  DataLoggingVariableName=ScopeData3
  Integrator : Integrator
  Multiply-Add2 : hdlsllib/HDL Operations/Multiply-Add  Function=c+(a.*b)  datatype=Inherit: Inherit via internal rule  DoSatur=off  FMA=off
  PS-Simulink Converter10 : nesl_utility/PS-Simulink Converter  PhysicalDomain=network_engine_domain  SubClassName=ps_output  LeftPortType=input  RightPortType=output  PseudoPeriodic=off  Frequencies=[]  VectorFormat=inherit  Unit=inherit  AffineConversion=off
  PS-Simulink Converter11 : nesl_utility/PS-Simulink Converter  PhysicalDomain=network_engine_domain  SubClassName=ps_output  LeftPortType=input  RightPortType=output  PseudoPeriodic=off  Frequencies=[]  VectorFormat=inherit  Unit=inherit  AffineConversion=off
  T_hip : PMIOPort  Side=Left
  w_hip : PMIOPort  Port=2  Side=Left
  Out1 : Outport
  wires:
  PS-Simulink Converter10/1 -> Multiply-Add2/1
  Integrator/1 -> Out1/1, Energy Wheel RR/1
  PS-Simulink Converter11/1 -> Multiply-Add2/2
  Constant/1 -> Multiply-Add2/3
  Abs/1 -> Integrator/1
  Multiply-Add2/1 -> Abs/1
  connections:
  T_hip/RConn1 -- PS-Simulink Converter11/LConn1
  w_hip/RConn1 -- PS-Simulink Converter10/LConn1

== system Trot/RR/Energy_RR/Energy_Knee ==
  Abs : Abs  SaturateOnIntegerOverflow=off
  Constant : Constant  Value=0
  Energy Wheel RR : Scope
      settings: ActiveDisplayYMinimum=-137.61876169666837  ActiveDisplayYMaximum=1238.5688552700155  DataLoggingVariableName=ScopeData3
  Integrator : Integrator
  Multiply-Add2 : hdlsllib/HDL Operations/Multiply-Add  Function=c+(a.*b)  datatype=Inherit: Inherit via internal rule  DoSatur=off  FMA=off
  PS-Simulink Converter10 : nesl_utility/PS-Simulink Converter  PhysicalDomain=network_engine_domain  SubClassName=ps_output  LeftPortType=input  RightPortType=output  PseudoPeriodic=off  Frequencies=[]  VectorFormat=inherit  Unit=inherit  AffineConversion=off
  PS-Simulink Converter11 : nesl_utility/PS-Simulink Converter  PhysicalDomain=network_engine_domain  SubClassName=ps_output  LeftPortType=input  RightPortType=output  PseudoPeriodic=off  Frequencies=[]  VectorFormat=inherit  Unit=inherit  AffineConversion=off
  T_knee : PMIOPort  Side=Left
  w_knee : PMIOPort  Port=2  Side=Left
  Out1 : Outport
  wires:
  Multiply-Add2/1 -> Abs/1
  Abs/1 -> Integrator/1
  Constant/1 -> Multiply-Add2/3
  PS-Simulink Converter11/1 -> Multiply-Add2/2
  Integrator/1 -> Energy Wheel RR/1, Out1/1
  PS-Simulink Converter10/1 -> Multiply-Add2/1
  connections:
  w_knee/RConn1 -- PS-Simulink Converter10/LConn1
  T_knee/RConn1 -- PS-Simulink Converter11/LConn1

== system Trot/RR/Energy_RR/Energy_Shoulder ==
  Abs : Abs  SaturateOnIntegerOverflow=off
  Constant : Constant  Value=0
  Energy Wheel RR : Scope
      settings: ActiveDisplayYMinimum=-137.61876169666837  ActiveDisplayYMaximum=1238.5688552700155  DataLoggingVariableName=ScopeData3
  Integrator : Integrator
  Multiply-Add2 : hdlsllib/HDL Operations/Multiply-Add  Function=c+(a.*b)  datatype=Inherit: Inherit via internal rule  DoSatur=off  FMA=off
  PS-Simulink Converter10 : nesl_utility/PS-Simulink Converter  PhysicalDomain=network_engine_domain  SubClassName=ps_output  LeftPortType=input  RightPortType=output  PseudoPeriodic=off  Frequencies=[]  VectorFormat=inherit  Unit=inherit  AffineConversion=off
  PS-Simulink Converter11 : nesl_utility/PS-Simulink Converter  PhysicalDomain=network_engine_domain  SubClassName=ps_output  LeftPortType=input  RightPortType=output  PseudoPeriodic=off  Frequencies=[]  VectorFormat=inherit  Unit=inherit  AffineConversion=off
  T_Shoulder : PMIOPort  Side=Left
  w_Shoulder : PMIOPort  Port=2  Side=Left
  Out1 : Outport
  wires:
  PS-Simulink Converter10/1 -> Multiply-Add2/1
  Integrator/1 -> Out1/1, Energy Wheel RR/1
  PS-Simulink Converter11/1 -> Multiply-Add2/2
  Constant/1 -> Multiply-Add2/3
  Abs/1 -> Integrator/1
  Multiply-Add2/1 -> Abs/1
  connections:
  T_Shoulder/RConn1 -- PS-Simulink Converter11/LConn1
  w_Shoulder/RConn1 -- PS-Simulink Converter10/LConn1

== matlab function Trot/RR/MATLAB Function3 ==
  data: t input; q_roll output; leg_id input; q_hip output; q_knee output
function [q_roll, q_hip, q_knee] = motion_walker_v8_extended(t, leg_id)
    % Trot gait — diagonal pairs move together
    %   Group A: RF(0) + LR(2)  phase = 0.0
    %   Group B: LF(1) + RR(3)  phase = 0.5
    
    % ================= Tunables =================
    ang_hip_crouch = deg2rad(30);    % Hip joint crouch angle maintained at 30 degrees
    ang_crouch     = deg2rad(-40);   % Knee joint crouch angle maintained at -40 degrees
    
    % <--- Modification 1: Reduce step size
    hip_swing_amp  = deg2rad(8);
    
    ang_fwd  = ang_hip_crouch - hip_swing_amp;  % 24 degrees
    ang_back = ang_hip_crouch + hip_swing_amp;  % 36 degrees
    
    % <--- Modification 2: Reduce auxiliary motion amplitude to match the smaller step size
    ang_lift       = deg2rad(-5);    % Leg lift bending reduced
    ang_comp       = deg2rad(-6);    % Stance phase compensation reduced
    
    % ================= Timing =================
    T_crouch = 2.0;              
    T_hold   = 3.0;              
    T_ramp   = 2.0;              
    
    % <--- Modification 3: Increase cycle time to make it slower/smoother
    T_cycle  = 1.8;
    duty     = 0.50;             
    
    % ================= Phase offsets =================
    phase_offset = [0.0, 0.5, 0.0, 0.5];
    phi = phase_offset(leg_id + 1);
    
    % ================= Smooth interpolators =================
    smooth = @(x) (1 - cos(x * pi)) / 2;
    bump   = @(x) (1 - cos(2 * x * pi)) / 2;
    
    % ==========================================================
    % Stage 1 & 2: Crouch & Hold
    % ==========================================================
    if t < T_crouch + T_hold
        s = smooth(min(t / T_crouch, 1.0));
        if t >= T_crouch
            s = 1.0;
        end
        q_roll = 0;                          
        q_hip  = s * ang_hip_crouch;
        q_knee = s * ang_crouch;
        return;
    end
    
    % ==========================================================
    % Stage 3: Trot
    % ==========================================================
    t_walk = t - T_crouch - T_hold;
    ramp = smooth(min(t_walk / T_ramp, 1.0));
    phase = mod(t_walk / T_cycle + phi, 1.0);
    
    % --- Full-amplitude trot trajectory ---
    if phase < duty
        % ===== STANCE: foot on ground =====
        % Keep your previously correct direction: ang_back -> ang_fwd
        s = smooth(phase / duty);
        hip_walk  = ang_back + s * (ang_fwd - ang_back); 
        
        % Knee joint compensation (amplitude reduced)
        knee_walk = ang_crouch + sin((phase / duty) * pi) * ang_comp;
        
    else
        % ===== SWING: foot in air =====
        % Keep your previously correct direction: ang_fwd -> ang_back
        s = (phase - duty) / (1.0 - duty);
        hip_walk  = ang_fwd + smooth(s) * (ang_back - ang_fwd);
        knee_walk = ang_crouch + bump(s) * ang_lift;
    end
    
    % --- Blend from rest into trot ---
    q_roll = 0;                              
    q_hip  = ang_hip_crouch + ramp * (hip_walk - ang_hip_crouch);
    q_knee = ang_crouch + ramp * (knee_walk - ang_crouch);
end

== matlab function Trot/FL/MATLAB Function3 ==
  data: t input; q_roll output; leg_id input; q_hip output; q_knee output
function [q_roll, q_hip, q_knee] = motion_walker_v8_extended(t, leg_id)
    % Trot gait — diagonal pairs move together
    %   Group A: RF(0) + LR(2)  phase = 0.0
    %   Group B: LF(1) + RR(3)  phase = 0.5
    
    % ================= Tunables =================
    ang_hip_crouch = deg2rad(30);    % Hip joint crouch angle maintained at 30 degrees
    ang_crouch     = deg2rad(-40);   % Knee joint crouch angle maintained at -40 degrees
    
    % <--- Modification 1: Reduce step size
    hip_swing_amp  = deg2rad(8);
    
    ang_fwd  = ang_hip_crouch - hip_swing_amp;  % 24 degrees
    ang_back = ang_hip_crouch + hip_swing_amp;  % 36 degrees
    
    % <--- Modification 2: Reduce auxiliary motion amplitude to match the smaller step size
    ang_lift       = deg2rad(-5);    % Leg lift bending reduced
    ang_comp       = deg2rad(-6);    % Stance phase compensation reduced
    
    % ================= Timing =================
    T_crouch = 2.0;              
    T_hold   = 3.0;              
    T_ramp   = 2.0;              
    
    % <--- Modification 3: Increase cycle time to make it slower/smoother
    T_cycle  = 1.8;
    duty     = 0.50;             
    
    % ================= Phase offsets =================
    phase_offset = [0.0, 0.5, 0.0, 0.5];
    phi = phase_offset(leg_id + 1);
    
    % ================= Smooth interpolators =================
    smooth = @(x) (1 - cos(x * pi)) / 2;
    bump   = @(x) (1 - cos(2 * x * pi)) / 2;
    
    % ==========================================================
    % Stage 1 & 2: Crouch & Hold
    % ==========================================================
    if t < T_crouch + T_hold
        s = smooth(min(t / T_crouch, 1.0));
        if t >= T_crouch
            s = 1.0;
        end
        q_roll = 0;                          
        q_hip  = s * ang_hip_crouch;
        q_knee = s * ang_crouch;
        return;
    end
    
    % ==========================================================
    % Stage 3: Trot
    % ==========================================================
    t_walk = t - T_crouch - T_hold;
    ramp = smooth(min(t_walk / T_ramp, 1.0));
    phase = mod(t_walk / T_cycle + phi, 1.0);
    
    % --- Full-amplitude trot trajectory ---
    if phase < duty
        % ===== STANCE: foot on ground =====
        % Keep your previously correct direction: ang_back -> ang_fwd
        s = smooth(phase / duty);
        hip_walk  = ang_back + s * (ang_fwd - ang_back); 
        
        % Knee joint compensation (amplitude reduced)
        knee_walk = ang_crouch + sin((phase / duty) * pi) * ang_comp;
        
    else
        % ===== SWING: foot in air =====
        % Keep your previously correct direction: ang_fwd -> ang_back
        s = (phase - duty) / (1.0 - duty);
        hip_walk  = ang_fwd + smooth(s) * (ang_back - ang_fwd);
        knee_walk = ang_crouch + bump(s) * ang_lift;
    end
    
    % --- Blend from rest into trot ---
    q_roll = 0;                              
    q_hip  = ang_hip_crouch + ramp * (hip_walk - ang_hip_crouch);
    q_knee = ang_crouch + ramp * (knee_walk - ang_crouch);
end

== matlab function Trot/FR/MATLAB Function3 ==
  data: t input; q_roll output; leg_id input; q_hip output; q_knee output
function [q_roll, q_hip, q_knee] = motion_walker_v8_extended(t, leg_id)
    % Trot gait — diagonal pairs move together
    %   Group A: RF(0) + LR(2)  phase = 0.0
    %   Group B: LF(1) + RR(3)  phase = 0.5
    
    % ================= Tunables =================
    ang_hip_crouch = deg2rad(30);    % Hip joint crouch angle maintained at 30 degrees
    ang_crouch     = deg2rad(-40);   % Knee joint crouch angle maintained at -40 degrees
    
    % <--- Modification 1: Reduce step size
    hip_swing_amp  = deg2rad(8);
    
    ang_fwd  = ang_hip_crouch - hip_swing_amp;  % 24 degrees
    ang_back = ang_hip_crouch + hip_swing_amp;  % 36 degrees
    
    % <--- Modification 2: Reduce auxiliary motion amplitude to match the smaller step size
    ang_lift       = deg2rad(-5);    % Leg lift bending reduced
    ang_comp       = deg2rad(-6);    % Stance phase compensation reduced
    
    % ================= Timing =================
    T_crouch = 2.0;              
    T_hold   = 3.0;              
    T_ramp   = 2.0;              
    
    % <--- Modification 3: Increase cycle time to make it slower/smoother
    T_cycle  = 1.8;
    duty     = 0.50;             
    
    % ================= Phase offsets =================
    phase_offset = [0.0, 0.5, 0.0, 0.5];
    phi = phase_offset(leg_id + 1);
    
    % ================= Smooth interpolators =================
    smooth = @(x) (1 - cos(x * pi)) / 2;
    bump   = @(x) (1 - cos(2 * x * pi)) / 2;
    
    % ==========================================================
    % Stage 1 & 2: Crouch & Hold
    % ==========================================================
    if t < T_crouch + T_hold
        s = smooth(min(t / T_crouch, 1.0));
        if t >= T_crouch
            s = 1.0;
        end
        q_roll = 0;                          
        q_hip  = s * ang_hip_crouch;
        q_knee = s * ang_crouch;
        return;
    end
    
    % ==========================================================
    % Stage 3: Trot
    % ==========================================================
    t_walk = t - T_crouch - T_hold;
    ramp = smooth(min(t_walk / T_ramp, 1.0));
    phase = mod(t_walk / T_cycle + phi, 1.0);
    
    % --- Full-amplitude trot trajectory ---
    if phase < duty
        % ===== STANCE: foot on ground =====
        % Keep your previously correct direction: ang_back -> ang_fwd
        s = smooth(phase / duty);
        hip_walk  = ang_back + s * (ang_fwd - ang_back); 
        
        % Knee joint compensation (amplitude reduced)
        knee_walk = ang_crouch + sin((phase / duty) * pi) * ang_comp;
        
    else
        % ===== SWING: foot in air =====
        % Keep your previously correct direction: ang_fwd -> ang_back
        s = (phase - duty) / (1.0 - duty);
        hip_walk  = ang_fwd + smooth(s) * (ang_back - ang_fwd);
        knee_walk = ang_crouch + bump(s) * ang_lift;
    end
    
    % --- Blend from rest into trot ---
    q_roll = 0;                              
    q_hip  = ang_hip_crouch + ramp * (hip_walk - ang_hip_crouch);
    q_knee = ang_crouch + ramp * (knee_walk - ang_crouch);
end
